simulink model "CruiseControl_harness_SLDV_final"  (R2015a)
settings: Solver=FixedStepDiscrete  StartTime=0.0  StopTime=2  FixedStep=0.1  RelTol=1e-3
PostLoadFcn:
  | CruiseControl_dd;
undefined symbols (not defined in the file): sigbuilder_block
libraries: simulink x1
settings Model: SldvGeneratedHarnessModel=TestUnitModel=CruiseControl|  CovMetricSettings=dcme  CovHTMLOptions=-aTS=1 -bRG=1 -bTC=0 -hTR=0 -nFC=0 -scm=1 -bcm=1  CovHtmlReporting=off  covSaveCumulativeToWorkspaceVar=off  CovSaveSingleToWorkspaceVar=off  CovModelRefEnable=off  CovExternalEMLEnable=on  Creator=The MathWorks Inc.  LastModifiedBy=colosky
settings DataIOCC: SaveFormat=StructureWithTime  SaveOutput=off  InspectSignalLogs=on  SaveTime=off
settings OptimizationCC: InlineParams=on  InlineInvariantSignals=on  ExpressionDepthLimit=2147483647  InitFltsAndDblsToZero=on  NoFixptDivByZeroProtection=on  OptimizeModelRefInitCode=on
settings DebuggingCC: SignalInfNanChecking=warning  SaveWithParameterizedLinksMsg=none  UnderspecifiedInitializationDetection=Classic  MergeDetectMultiDrivingBlocksExec=none  SolverPrmCheckMsg=warning  InheritedTsInSrcMsg=none  FcnCallInpInsideContextMsg=UseLocalSettings  UniqueDataStoreMsg=warning  StateNameClashWarn=warning  StrictBusMsg=ErrorOnBusTreatedAsVector
settings ModelReferenceCC: ModelReferenceNumInstancesAllowed=Single
settings SFSimCC: SimParseCustomCode=off
settings RTWCC: SystemTargetFile=ert.tlc  TemplateMakefile=ert_default_tmf  Description=Embedded Coder  GenerateReport=on  IncludeHyperlinkInReport=on  LaunchReport=on  PortableWordSizes=on  GenerateTraceInfo=on  GenerateTraceReport=on  GenerateTraceReportSl=on  GenerateTraceReportSf=on  GenerateTraceReportEml=on
settings CodeAppCC: IgnoreCustomStorageClasses=off  CustomSymbolStrGlobalVar=$N$M
settings ERTTargetCC: ParMdlRefBuildCompliant=on  CompOptLevelCompliant=on  ConcurrentExecutionCompliant=on  ERTFirstTimeCompliant=on  SupportContinuousTime=off  SupportVariableSizeSignals=off  ModelStepFunctionPrototypeControlCompliant=on  CPPClassGenCompliant=on  ERTCustomFileTemplate=example_file_process.tlc
settings ConfigComp: Description=Design Verifier Custom Configuration Component  DVMode=DesignErrorDetection  DVMaxProcessTime=3000  DVDisplayUnsatisfiableObjectives=on  DVAutomaticStubbing=off  DVMakeOutputFilesUnique=off  DVParameters=on  DVParametersUseConfig=on  DVModelCoverageObjectives=MCDC  DVMaxTestCaseSteps=500  DVTestSuiteOptimization=CombinedObjectives  DVAssertions=EnableAll  DVProofAssumptions=EnableAll  DVIgnoreCovSatisfied=on  DVCoverageDataFile=CruiseControlCovManual.cvt  DVDetectIntegerOverflow=off  DVDetectDeadLogic=on  DVDetectActiveLogic=on  DVMaxViolationSteps=50  DVSaveDataFile=off  DVSaveHarnessModel=on  DVHarnessModelFileName=$ModelName$_harness_SLDV  DVReportIncludeGraphics=on  PSAutoStubLUT=off

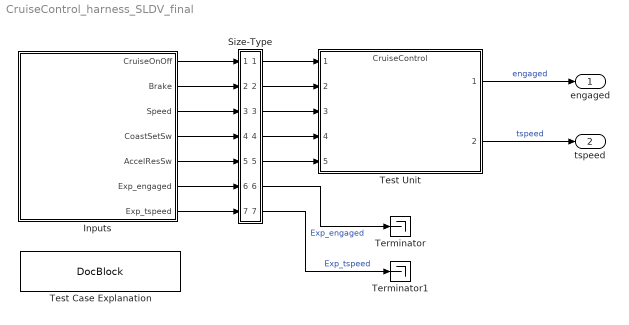
== system CruiseControl_harness_SLDV_final ==
  Inputs : Subsystem  Tag=STV Subsys  LoadFcn=sigbuilder_block('load',[-57 207 427.2 345.6 ]);  StartFcn=sigbuilder_block('start');  StopFcn=sigbuilder_block('stop');  ClipboardFcn=sigbuilder_block('clipboard');  mask(Sigbuilder block){}
      mask init:
      | if ~strcmp(get_param(bdroot(gcb),'SimulationStatus'),'stopped'),tuvar = sigbuilder_block('maskInit'); end
      settings: CopyFcn=sigbuilder_block('copy');  DeleteFcn=sigbuilder_block('delete');  ModelCloseFcn=sigbuilder_block('modelClose');  PreSaveFcn=sigbuilder_block('preSave');  PauseFcn=sigbuilder_block('pause');  ContinueFcn=sigbuilder_block('continue');  NameChangeFcn=sigbuilder_block('namechange');  OpenFcn=sigbuilder_block('open');  CloseFcn=sigbuilder_block('close');
      mask Display: plot(0, 0, 100, 100,[2, 2, 32, 32, 2], [68, 8, 8, 68, 68],[32, 2], [38, 38], [32, 19, 2],[53, 60, 44], [32, 17, 17, 2],[16, 16, 31, 31]);txt = getActiveGroup(gcbh);text(2, 100, txt,'verticalAlignment', 'top');
  Size-Type : Subsystem
  Terminator : Terminator
  Terminator1 : Terminator
  Test Case Explanation : simulink/Model-Wide Utilities/DocBlock  DocumentType=Text
  Test Unit : ModelReference  ModelNameDialog=CruiseControl  SimulationMode=Normal  ModelReferenceVersion=1.450  CopyOfModelName=CruiseControl
  engaged : Outport
  tspeed : Outport  Port=2
  wires:
  Size-Type/1(Out1) -> Test Unit/1
  Size-Type/2(Out2) -> Test Unit/2
  Size-Type/3(Out3) -> Test Unit/3
  Size-Type/4(Out4) -> Test Unit/4
  Size-Type/5(Out5) -> Test Unit/5
  Test Unit/1 -> engaged/1  "engaged"
  Test Unit/2 -> tspeed/1  "tspeed"
  Inputs/5(AccelResSw) -> Size-Type/5(In5)
  Inputs/4(CoastSetSw) -> Size-Type/4(In4)
  Inputs/7(Exp_tspeed) -> Size-Type/7(In7)
  Inputs/6(Exp_engaged) -> Size-Type/6(In6)
  Inputs/3(Speed) -> Size-Type/3(In3)
  Inputs/2(Brake) -> Size-Type/2(In2)
  Inputs/1(CruiseOnOff) -> Size-Type/1(In1)
  Size-Type/6(Out6) -> Terminator/1  "Exp_engaged"
  Size-Type/7(Out7) -> Terminator1/1  "Exp_tspeed"

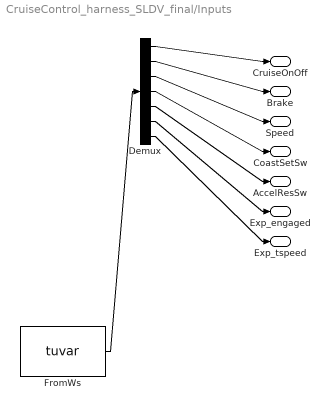
== system CruiseControl_harness_SLDV_final/Inputs ==
  Demux : Demux  Tag=STV Demux  Outputs=7
  FromWs : FromWorkspace  Tag=STV FromWs  VariableName=tuvar  SampleTime=0
      SigBuilderData=|
      | dataSet(1).timeRange = [0 2]
      | dataSet(1).name = 'Init Not Enable or Engaged'
      | dataSet(2).timeRange = [0 2]
      | dataSet(2).name = 'Not Engaged with Enable'
      | dataSet(3).timeRange = [0 2]
      | dataSet(3).name = 'Disengage with Disable'
      | dataSet(4).timeRange = [0 2]
      | dataSet(4).name = 'Engage 1st with CoastSetSW'
      | dataSet(5).timeRange = [0 2]
      | dataSet(5).name = 'No Engage 1st with AccelResSW'
      | dataSet(6).timeRange = [0 2]
      | dataSet(6).name = 'Disengage with Brake'
      | sbobj.Name = 'Signal Builder'
      | sbobj.Groups(1).Name = 'Init Not Enable or Engaged'
      | sbobj.Groups(1).Signals(1).Name = 'CruiseOnOff'
      | sbobj.Groups(1).Signals(1).XData = [0 1 2]
      | sbobj.Groups(1).Signals(1).YData = [0 0 0]
      | sbobj.Groups(1).Signals(2).Name = 'Brake'
      | sbobj.Groups(1).Signals(2).XData = [0 1 2]
      | sbobj.Groups(1).Signals(2).YData = [0 0 0]
      | sbobj.Groups(1).Signals(3).Name = 'Speed'
      | sbobj.Groups(1).Signals(3).XData = [0 1 2]
      | sbobj.Groups(1).Signals(3).YData = [50 50 50]
      | sbobj.Groups(1).Signals(4).Name = 'CoastSetSw'
      | sbobj.Groups(1).Signals(4).XData = [0 1 2]
      | sbobj.Groups(1).Signals(4).YData = [0 0 0]
      | sbobj.Groups(1).Signals(5).Name = 'AccelResSw'
      | sbobj.Groups(1).Signals(5).XData = [0 1 2]
      | sbobj.Groups(1).Signals(5).YData = [0 0 0]
      | sbobj.Groups(1).Signals(6).Name = 'Exp_engaged'
      | sbobj.Groups(1).Signals(6).XData = [0 1 2]
      | sbobj.Groups(1).Signals(6).YData = [0 0 0]
      | sbobj.Groups(1).Signals(7).Name = 'Exp_tspeed'
      | sbobj.Groups(1).Signals(7).XData = [0 1 2]
      | sbobj.Groups(1).Signals(7).YData = [0 0 0]
      | sbobj.Groups(1).TimeRange = [0 2]
      | sbobj.Groups(2).Name = 'Not Engaged with Enable'
      | sbobj.Groups(2).Signals(1).Name = 'CruiseOnOff'
      | sbobj.Groups(2).Signals(1).XData = [0 1 1 2]
      | sbobj.Groups(2).Signals(1).YData = [0 0 1 1]
      | sbobj.Groups(2).Signals(2).Name = 'Brake'
      | sbobj.Groups(2).Signals(2).XData = [0 1 2]
      | sbobj.Groups(2).Signals(2).YData = [0 0 0]
      | sbobj.Groups(2).Signals(3).Name = 'Speed'
      | sbobj.Groups(2).Signals(3).XData = [0 1 2]
      | sbobj.Groups(2).Signals(3).YData = [0 0 0]
      | sbobj.Groups(2).Signals(4).Name = 'CoastSetSw'
      | sbobj.Groups(2).Signals(4).XData = [0 1 2]
      | sbobj.Groups(2).Signals(4).YData = [0 0 0]
      | sbobj.Groups(2).Signals(5).Name = 'AccelResSw'
      | sbobj.Groups(2).Signals(5).XData = [0 1 2]
      | sbobj.Groups(2).Signals(5).YData = [0 0 0]
      | sbobj.Groups(2).Signals(6).Name = 'Exp_engaged'
      | sbobj.Groups(2).Signals(6).XData = [0 1 2]
      | sbobj.Groups(2).Signals(6).YData = [0 0 0]
      | sbobj.Groups(2).Signals(7).Name = 'Exp_tspeed'
      | sbobj.Groups(2).Signals(7).XData = [0 1 2]
      | sbobj.Groups(2).Signals(7).YData = [0 0 0]
      | sbobj.Groups(2).TimeRange = [0 2]
      | sbobj.Groups(3).Name = 'Disengage with Disable'
      | sbobj.Groups(3).Signals(1).Name = 'CruiseOnOff'
      | sbobj.Groups(3).Signals(1).XData = [0 0.5 0.5 1 1.1 1.5 1.5 2]
      | sbobj.Groups(3).Signals(1).YData = [0 0 1 1 1 1 0 0]
      | sbobj.Groups(3).Signals(2).Name = 'Brake'
      | sbobj.Groups(3).Signals(2).XData = [0 0.5 1 1.1 1.5 2]
      | sbobj.Groups(3).Signals(2).YData = [0 0 0 0 0 0]
      | sbobj.Groups(3).Signals(3).Name = 'Speed'
      | sbobj.Groups(3).Signals(3).XData = [0 0.5 1 1.1 1.5 2]
      | sbobj.Groups(3).Signals(3).YData = [50 50 50 50 50 50]
      | sbobj.Groups(3).Signals(4).Name = 'CoastSetSw'
      | sbobj.Groups(3).Signals(4).XData = [0 0.5 1 1 1.1 1.1 1.5 2]
      | sbobj.Groups(3).Signals(4).YData = [0 0 0 1 1 0 0 0]
      | sbobj.Groups(3).Signals(5).Name = 'AccelResSw'
      | sbobj.Groups(3).Signals(5).XData = [0 0.5 1 1.1 1.5 2]
      | sbobj.Groups(3).Signals(5).YData = [0 0 0 0 0 0]
      | sbobj.Groups(3).Signals(6).Name = 'Exp_engaged'
      | sbobj.Groups(3).Signals(6).XData = [0 0.5 1 1 1.1 1.5 1.5 2]
      | sbobj.Groups(3).Signals(6).YData = [0 0 0 1 1 1 0 0]
      | sbobj.Groups(3).Signals(7).Name = 'Exp_tspeed'
      | sbobj.Groups(3).Signals(7).XData = [0 0.5 1 1 1.1 1.5 1.5 2]
      | sbobj.Groups(3).Signals(7).YData = [0 0 0 50 50 50 0 0]
      | sbobj.Groups(3).TimeRange = [0 2]
      | sbobj.Groups(4).Name = 'Engage 1st with CoastSetSW'
      | sbobj.Groups(4).Signals(1).Name = 'CruiseOnOff'
      | sbobj.Groups(4).Signals(1).XData = [0 0.5 0.5 1 1.1 2]
      | sbobj.Groups(4).Signals(1).YData = [0 0 1 1 1 1]
      | sbobj.Groups(4).Signals(2).Name = 'Brake'
      | sbobj.Groups(4).Signals(2).XData = [0 0.5 1 1.1 2]
      | sbobj.Groups(4).Signals(2).YData = [0 0 0 0 0]
      | sbobj.Groups(4).Signals(3).Name = 'Speed'
      | sbobj.Groups(4).Signals(3).XData = [0 0.5 1 1.1 2]
      | sbobj.Groups(4).Signals(3).YData = [50 50 50 50 50]
      | sbobj.Groups(4).Signals(4).Name = 'CoastSetSw'
      | sbobj.Groups(4).Signals(4).XData = [0 0.5 1 1 1.1 1.1 2]
      | sbobj.Groups(4).Signals(4).YData = [0 0 0 1 1 0 0]
      | sbobj.Groups(4).Signals(5).Name = 'AccelResSw'
      | sbobj.Groups(4).Signals(5).XData = [0 0.5 1 1.1 2]
      | sbobj.Groups(4).Signals(5).YData = [0 0 0 0 0]
      | sbobj.Groups(4).Signals(6).Name = 'Exp_engaged'
      | sbobj.Groups(4).Signals(6).XData = [0 0.5 1 1 1.1 2]
      | sbobj.Groups(4).Signals(6).YData = [0 0 0 1 1 1]
      | sbobj.Groups(4).Signals(7).Name = 'Exp_tspeed'
      | sbobj.Groups(4).Signals(7).XData = [0 0.5 1 1 1.1 2]
      | sbobj.Groups(4).Signals(7).YData = [0 0 0 50 50 50]
      | sbobj.Groups(4).TimeRange = [0 2]
      | sbobj.Groups(5).Name = 'No Engage 1st with AccelResSW'
      | sbobj.Groups(5).Signals(1).Name = 'CruiseOnOff'
      | sbobj.Groups(5).Signals(1).XData = [0 0.5 0.5 1 1.1 2]
      | sbobj.Groups(5).Signals(1).YData = [0 0 1 1 1 1]
      | sbobj.Groups(5).Signals(2).Name = 'Brake'
      | sbobj.Groups(5).Signals(2).XData = [0 0.5 1 1.1 2]
      | sbobj.Groups(5).Signals(2).YData = [0 0 0 0 0]
      | sbobj.Groups(5).Signals(3).Name = 'Speed'
      | sbobj.Groups(5).Signals(3).XData = [0 0.5 1 1.1 2]
      | sbobj.Groups(5).Signals(3).YData = [50 50 50 50 50]
      | sbobj.Groups(5).Signals(4).Name = 'CoastSetSw'
      | sbobj.Groups(5).Signals(4).XData = [0 0.5 1 1.1 2]
      | sbobj.Groups(5).Signals(4).YData = [0 0 0 0 0]
      | sbobj.Groups(5).Signals(5).Name = 'AccelResSw'
      | sbobj.Groups(5).Signals(5).XData = [0 0.5 1 1 1.1 1.1 2]
      | sbobj.Groups(5).Signals(5).YData = [0 0 0 1 1 0 0]
      | sbobj.Groups(5).Signals(6).Name = 'Exp_engaged'
      | sbobj.Groups(5).Signals(6).XData = [0 0.5 1 1.1 2]
      | sbobj.Groups(5).Signals(6).YData = [0 0 0 0 0]
      | sbobj.Groups(5).Signals(7).Name = 'Exp_tspeed'
      | sbobj.Groups(5).Signals(7).XData = [0 0.5 1 1.1 2]
      | sbobj.Groups(5).Signals(7).YData = [0 0 0 0 0]
      | sbobj.Groups(5).TimeRange = [0 2]
      | sbobj.Groups(6).Name = 'Disengage with Brake'
      | sbobj.Groups(6).Signals(1).Name = 'CruiseOnOff'
      | sbobj.Groups(6).Signals(1).XData = [0 0.5 0.5 1 1.1 1.5 1.6 2]
      | sbobj.Groups(6).Signals(1).YData = [0 0 1 1 1 1 1 1]
      | sbobj.Groups(6).Signals(2).Name = 'Brake'
      | sbobj.Groups(6).Signals(2).XData = [0 0.5 1 1.1 1.5 1.5 1.6 1.6 2]
      | sbobj.Groups(6).Signals(2).YData = [0 0 0 0 0 1 1 0 0]
      | sbobj.Groups(6).Signals(3).Name = 'Speed'
      | sbobj.Groups(6).Signals(3).XData = [0 0.5 1 1.1 1.5 1.6 2]
      | sbobj.Groups(6).Signals(3).YData = [50 50 50 50 50 50 50]
      | sbobj.Groups(6).Signals(4).Name = 'CoastSetSw'
      | sbobj.Groups(6).Signals(4).XData = [0 0.5 1 1 1.1 1.1 1.5 1.6 2]
      | sbobj.Groups(6).Signals(4).YData = [0 0 0 1 1 0 0 0 0]
      | sbobj.Groups(6).Signals(5).Name = 'AccelResSw'
      | sbobj.Groups(6).Signals(5).XData = [0 0.5 1 1.1 1.5 1.6 2]
      | sbobj.Groups(6).Signals(5).YData = [0 0 0 0 0 0 0]
      | sbobj.Groups(6).Signals(6).Name = 'Exp_engaged'
      | sbobj.Groups(6).Signals(6).XData = [0 0.5 1 1 1.1 1.5 1.5 1.6 2]
      | sbobj.Groups(6).Signals(6).YData = [0 0 0 1 1 1 0 0 0]
      | sbobj.Groups(6).Signals(7).Name = 'Exp_tspeed'
      | sbobj.Groups(6).Signals(7).XData = [0 0.5 1 1 1.1 1.5 1.6 2]
      | sbobj.Groups(6).Signals(7).YData = [0 0 0 50 50 50 50 50]
      | sbobj.Groups(6).TimeRange = [0 2]
  CruiseOnOff : Outport
  Brake : Outport  Tag=STV Outport  Port=2
  Speed : Outport  Tag=STV Outport  Port=3
  CoastSetSw : Outport  Tag=STV Outport  Port=4
  AccelResSw : Outport  Tag=STV Outport  Port=5
  Exp_engaged : Outport  Tag=STV Outport  Port=6
  Exp_tspeed : Outport  Tag=STV Outport  Port=7
  wires:
  FromWs/1 -> Demux/1
  Demux/1 -> CruiseOnOff/1
  Demux/2 -> Brake/1
  Demux/3 -> Speed/1
  Demux/4 -> CoastSetSw/1
  Demux/5 -> AccelResSw/1
  Demux/6 -> Exp_engaged/1
  Demux/7 -> Exp_tspeed/1

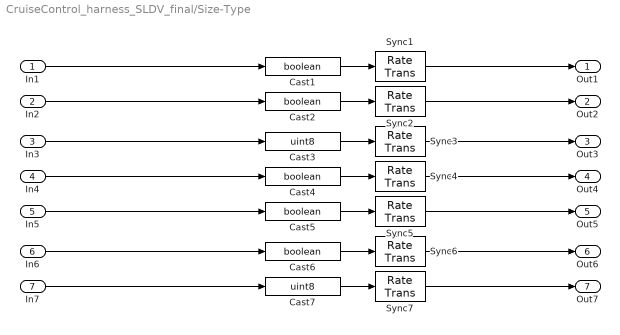
== system CruiseControl_harness_SLDV_final/Size-Type ==
  In1 : Inport
  In2 : Inport  Port=2
  In3 : Inport  Port=3
  In4 : Inport  Port=4
  In5 : Inport  Port=5
  In6 : Inport  Port=6
  In7 : Inport  Port=7
  Cast{1..2,4..6} (5 alike) : DataTypeConversion  OutDataTypeStr=boolean  RndMeth=Nearest  SaturateOnIntegerOverflow=on
  Cast3 : DataTypeConversion  OutDataTypeStr=uint8  RndMeth=Nearest  SaturateOnIntegerOverflow=on
  Cast7 : DataTypeConversion  OutDataTypeStr=uint8  RndMeth=Nearest  SaturateOnIntegerOverflow=on
  Sync{1..7} (7 alike) : RateTransition  OutPortSampleTime=[0.10000000000000001,0]
  Out1 : Outport
  Out2 : Outport  Port=2
  Out3 : Outport  Port=3
  Out4 : Outport  Port=4
  Out5 : Outport  Port=5
  Out6 : Outport  Port=6
  Out7 : Outport  Port=7
  wires:
  In1/1 -> Cast1/1
  Cast1/1 -> Sync1/1
  Sync1/1 -> Out1/1
  In2/1 -> Cast2/1
  Cast2/1 -> Sync2/1
  Sync2/1 -> Out2/1
  In3/1 -> Cast3/1
  Cast3/1 -> Sync3/1
  Sync3/1 -> Out3/1
  In4/1 -> Cast4/1
  Cast4/1 -> Sync4/1
  Sync4/1 -> Out4/1
  In5/1 -> Cast5/1
  Cast5/1 -> Sync5/1
  Sync5/1 -> Out5/1
  In6/1 -> Cast6/1
  Cast6/1 -> Sync6/1
  Sync6/1 -> Out6/1
  In7/1 -> Cast7/1
  Cast7/1 -> Sync7/1
  Sync7/1 -> Out7/1
